simulink model "QC_model"  (R2020a)
settings: Solver=ode5  StartTime=0.0  StopTime=10  FixedStep=basic_time_step  RelTol=1e-3  EnableMultiTasking=on
values from neighbouring files (symbols this model uses):
  b_hat_0 = [0;0;0]    [init.m]
  basic_time_step = 0.001    [init.m]
  e_g = [0;0;1]    [init.m]
  e_m = [1;0;0]    [init.m]
  Eul_hat_0 = [0;0;0]    [init.m]
  g = 9.81    [init.m]
  I = 0.025*eye(3)    [init.m]
  I_inv = inv(I)    [init.m]
  IMU_time_step = 0.002    [init.m]
  k1 = 1    [init.m]
  k2 = 1    [init.m]
  k_I = 10    [init.m]
  k_m = 200    [init.m]
  k_P = 5    [init.m]
  kd = [0.8 0 0 ... (first row only)    [init.m]
  KDP = 2    [init.m]
  KDR = 5    [init.m]
  KDY = 5    [init.m]
  ki = 0*[1.45 0 0 ... (first row only)    [init.m]
  kp = [0.7 0 0 ... (first row only)    [init.m]
  KPP = 35    [init.m]
  KPR = 35    [init.m]
  KPY = 35    [init.m]
  m = 1.5    [init.m]
  m0 = m*1    (= 1.5)    [init.m]
  max_pitch = sin(15*pi/180)    [init.m]
  max_roll = sin(15*pi/180)    [init.m]
  omega_0 = [0 0 0]    [init.m]
  omega_bias = 0*[0.01;-0.005;0.005]    [init.m]
  p_0 = [0 0 0]    [init.m]
  R_0 = eye(3)    [init.m]
  T_act_inv = inv(T_act)    [init.m]
  V_0 = [0 0 0]    [init.m]
  VICON_time_step = 0.016    [init.m]
  w_0 = 0*[1 1 1 1]    [init.m]
  w_max = [inf inf inf inf].^2    [init.m]
  w_min = [0 0 0 0]    [init.m]
undefined symbols (not defined in the file or in its folder): DiscIntNeverNeededParam, q_0
libraries: cstblocks x3, vrlib x2, simulink x1
settings Model: Creator=robu_pa  LastModifiedBy=RyllM
settings DataIOCC: LimitDataPoints=on  SaveFormat=Array  SignalLoggingSaveFormat=ModelDataLogs  ReturnWorkspaceOutputs=off
settings OptimizationCC: ExpressionDepthLimit=2147483647  LifeSpan=inf
settings DebuggingCC: UnderspecifiedInitializationDetection=Classic  MergeDetectMultiDrivingBlocksExec=none  SolverPrmCheckMsg=warning  FcnCallInpInsideContextMsg=warning  StateNameClashWarn=warning  SFUnexpectedBacktrackingDiag=warning  SFNoUnconditionalDefaultTransitionDiag=warning  SFExecutionAtInitializationDiag=none  ArithmeticOperatorsInVariantConditions=warning
settings HardwareCC: ProdBitPerPointer=32  ProdBitPerSizeT=32  ProdBitPerPtrDiffT=32  ProdLargestAtomicFloat=None  ProdIntDivRoundTo=Undefined  ProdEndianess=Unspecified  ProdWordSize=32  ProdHWDeviceType=32-bit Generic
settings ModelReferenceCC: PropagateSignalLabelsOutOfModel=off
settings SFSimCC: SimUseLocalCustomCode=off  CustomCodeUndefinedFunction=UseInterfaceOnly
settings RTWCC: Description=Linux Soft Real-Time Target  SystemTargetFile=lnx.tlc  MakeCommand=make_lnx  TemplateMakefile=lnx_unix.tmf  RTWUseLocalCustomCode=off
settings CodeAppCC: StateflowObjectComments=on
settings STFCustomTargetCC: ModelReferenceCompliant=off  MatFileLogging=on  CPPClassGenCompliant=on  GRTInterface=on  SystemTargetFile=lnx.tlc
settings GRTTargetCC: TargetLangStandard=C89/C90 (ANSI)  ModelReferenceCompliant=off  ParMdlRefBuildCompliant=off  CompOptLevelCompliant=off  ConcurrentExecutionCompliant=off  CombineOutputUpdateFcns=off  GRTInterface=on  UseToolchainInfoCompliant=off  ExtModeMexFile=noextcomm
settings ConfigComp: CovMetricSettings=dw  CovHtmlReporting=on  CovSaveCumulativeToWorkspaceVar=on  CovSaveSingleToWorkspaceVar=on  CovExternalEMLEnable=off

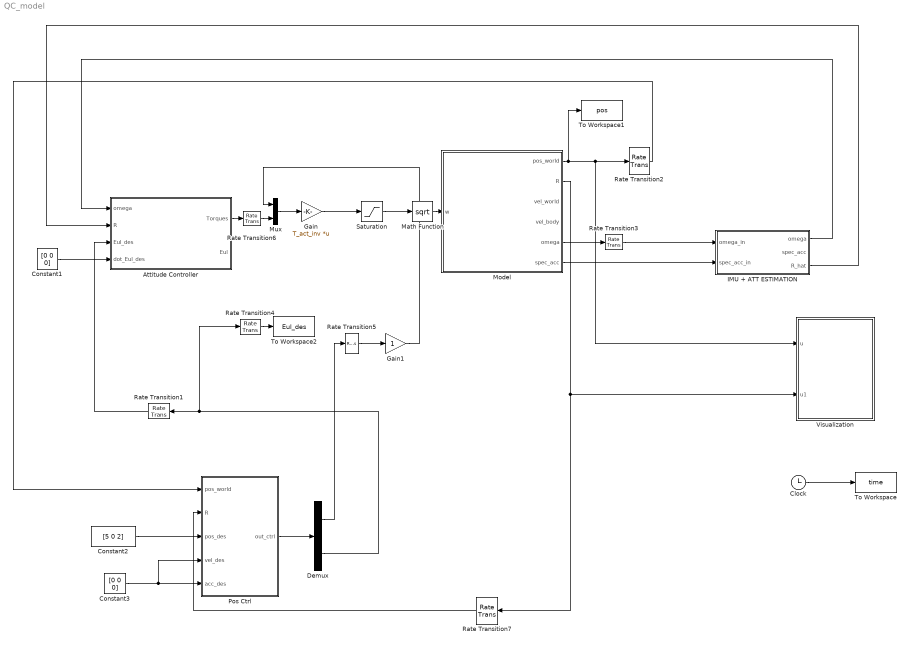
== system QC_model ==
  Attitude Controller : Subsystem  TreatAsAtomicUnit=on  SystemSampleTime=IMU_time_step
  Clock : Clock
  Constant1 : Constant  Value=[0 0 0]
  Constant2 : Constant  Value=[5 0 2]
  Constant3 : Constant  Value=[0 0 0]
  Demux : Demux  Outputs=[1 3]
  Gain : Gain  Gain=T_act_inv  Multiplication=Matrix(K*u)
  Gain1 : Gain
  IMU + ATT ESTIMATION : Subsystem  TreatAsAtomicUnit=on  SystemSampleTime=IMU_time_step
  Math Function : Math  Operator=sqrt  SignedPower=on  SaturateOnIntegerOverflow=on
  Model : Subsystem
  Mux : Mux  Inputs=2
  Pos Ctrl : Subsystem  TreatAsAtomicUnit=on  SystemSampleTime=VICON_time_step
  Rate Transition{1..7} (7 alike) : RateTransition
  Saturation : Saturate  UpperLimit=w_max  LowerLimit=w_min
  To Workspace : ToWorkspace  VariableName=time  SampleTime=-1
  To Workspace1 : ToWorkspace  VariableName=pos  SampleTime=-1
  To Workspace2 : ToWorkspace  VariableName=Eul_des  SampleTime=basic_time_step
  Visualization : Subsystem
  wires:
  Gain/1 -> Saturation/1
  Model/1(pos_world) -> To Workspace1/1, Visualization/1(u), Rate Transition2/1
  Model/6(spec_acc) -> IMU + ATT ESTIMATION/2(spec_acc_in)
  Model/5(omega) -> Rate Transition3/1
  Mux/1 -> Gain/1
  Attitude Controller/1(Torques) -> Rate Transition6/1
  Constant1/1 -> Attitude Controller/4(dot_Eul_des)
  Math Function/1 -> Model/1(w)
  Saturation/1 -> Math Function/1
  Rate Transition2/1 -> Pos Ctrl/1(pos_world)
  Demux/2 -> Rate Transition1/1, Rate Transition4/1
  Constant3/1 -> Pos Ctrl/5(acc_des), Pos Ctrl/4(vel_des)
  Pos Ctrl/1(out_ctrl) -> Demux/1
  Demux/1 -> Rate Transition5/1
  Rate Transition5/1 -> Gain1/1
  Gain1/1 -> Mux/1
  Rate Transition1/1 -> Attitude Controller/3(Eul_des)
  Model/2(R) -> Rate Transition7/1, Visualization/2(u1)
  Rate Transition6/1 -> Mux/2
  Rate Transition3/1 -> IMU + ATT ESTIMATION/1(omega_in)
  Rate Transition4/1 -> To Workspace2/1
  IMU + ATT ESTIMATION/1(omega) -> Attitude Controller/1(omega)
  IMU + ATT ESTIMATION/3(R_hat) -> Attitude Controller/2(R)
  Constant2/1 -> Pos Ctrl/3(pos_des)
  Rate Transition7/1 -> Pos Ctrl/2(R)
  Clock/1 -> To Workspace/1

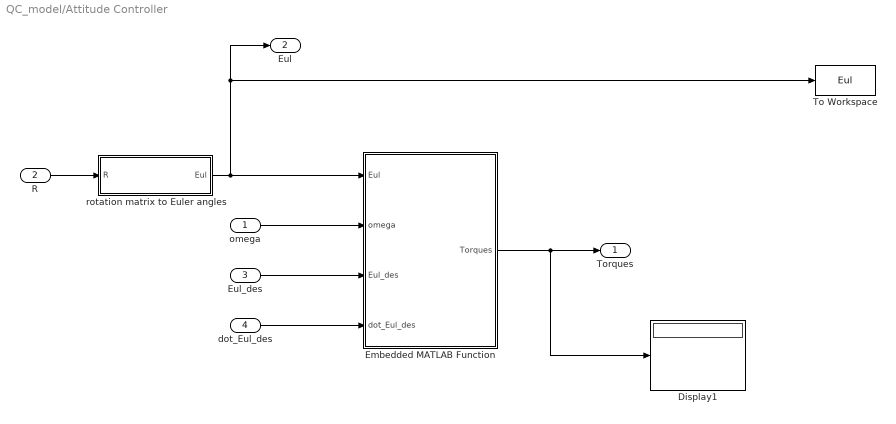
== system QC_model/Attitude Controller ==
  omega : Inport
  R : Inport  Port=2
  Eul_des : Inport  Port=3
  dot_Eul_des : Inport  Port=4
  Display1 : Display
  Embedded MATLAB Function : MATLAB Function  TreatAsAtomicUnit=on
  To Workspace : ToWorkspace  VariableName=Eul  SampleTime=-1
  rotation matrix to Euler angles : MATLAB Function  TreatAsAtomicUnit=on
  Torques : Outport  VectorParamsAs1DForOutWhenUnconnected=off
  Eul : Outport  Port=2  VectorParamsAs1DForOutWhenUnconnected=off
  wires:
  R/1 -> rotation matrix to Euler angles/1(R)
  rotation matrix to Euler angles/1(Eul) -> Embedded MATLAB Function/1(Eul), Eul/1, To Workspace/1
  omega/1 -> Embedded MATLAB Function/2(omega)
  Eul_des/1 -> Embedded MATLAB Function/3(Eul_des)
  dot_Eul_des/1 -> Embedded MATLAB Function/4(dot_Eul_des)
  Embedded MATLAB Function/1(Torques) -> Torques/1, Display1/1

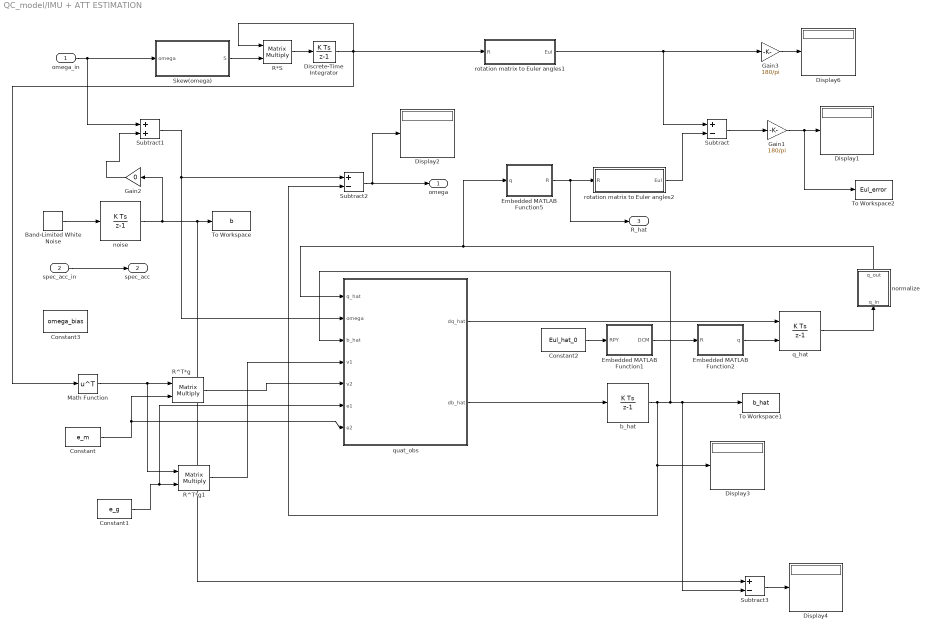
== system QC_model/IMU + ATT ESTIMATION ==
  omega_in : Inport
  spec_acc_in : Inport  Port=2
  Band-Limited White Noise : simulink/Sources/Band-Limited White Noise  Cov=[.0001 .0001 .0001]  Ts=IMU_time_step  seed=[23341 453 123]
  Constant : Constant  Value=e_m
  Constant1 : Constant  Value=e_g
  Constant2 : Constant  Value=Eul_hat_0
  Constant3 : Constant  Value=omega_bias
  Discrete-Time Integrator : DiscreteIntegrator  InitialCondition=R_0  SampleTime=-1  ICPrevOutput=DiscIntNeverNeededParam  ICPrevScaledInput=DiscIntNeverNeededParam
  Display{1..4,6} (5 alike) : Display
  Embedded MATLAB Function1 : MATLAB Function  TreatAsAtomicUnit=on
  Embedded MATLAB Function2 : MATLAB Function  TreatAsAtomicUnit=on
  Embedded MATLAB Function5 : MATLAB Function  TreatAsAtomicUnit=on
  Gain1 : Gain  Gain=180/pi
  Gain2 : Gain  Gain=0
  Gain3 : Gain  Gain=180/pi
  Math Function : Math  Operator=transpose  SignedPower=on  SaturateOnIntegerOverflow=on
  R*S : Product  Multiplication=Matrix(*)  RndMeth=Zero
  R^T*g : Product  Multiplication=Matrix(*)  RndMeth=Zero
  R^T*g1 : Product  Multiplication=Matrix(*)  RndMeth=Zero
  Skew(omega) : MATLAB Function  TreatAsAtomicUnit=on
  Subtract : Sum  Inputs=+-
  Subtract1 : Sum
  Subtract2 : Sum  Inputs=+-
  Subtract3 : Sum  Inputs=+-
  To Workspace : ToWorkspace  VariableName=b  SampleTime=-1
  To Workspace1 : ToWorkspace  VariableName=b_hat  SampleTime=-1
  To Workspace2 : ToWorkspace  VariableName=Eul_error  SampleTime=-1
  b_hat : DiscreteIntegrator  InitialCondition=b_hat_0  SampleTime=-1  ICPrevOutput=DiscIntNeverNeededParam  ICPrevScaledInput=DiscIntNeverNeededParam
  noise : DiscreteIntegrator  InitialCondition=b_hat_0  SampleTime=-1  ICPrevOutput=DiscIntNeverNeededParam  ICPrevScaledInput=DiscIntNeverNeededParam
  normalize : MATLAB Function  TreatAsAtomicUnit=on
  q_hat : DiscreteIntegrator  InitialConditionSource=external  InitialCondition=q_0  SampleTime=-1  ICPrevOutput=DiscIntNeverNeededParam  ICPrevScaledInput=DiscIntNeverNeededParam
  quat_obs : MATLAB Function  TreatAsAtomicUnit=on
  rotation matrix to Euler angles1 : MATLAB Function  TreatAsAtomicUnit=on
  rotation matrix to Euler angles2 : MATLAB Function  TreatAsAtomicUnit=on
  omega : Outport  VectorParamsAs1DForOutWhenUnconnected=off
  spec_acc : Outport  Port=2  VectorParamsAs1DForOutWhenUnconnected=off
  R_hat : Outport  Port=3  VectorParamsAs1DForOutWhenUnconnected=off
  wires:
  spec_acc_in/1 -> spec_acc/1
  omega_in/1 -> Skew(omega)/1(omega), Subtract1/1
  R*S/1 -> Discrete-Time Integrator/1
  Discrete-Time Integrator/1 -> Math Function/1, R*S/1, rotation matrix to Euler angles1/1(R)
  Skew(omega)/1(S) -> R*S/2
  rotation matrix to Euler angles1/1(Eul) -> Gain3/1, Subtract/1
  Gain3/1 -> Display6/1
  Math Function/1 -> R^T*g/1, R^T*g1/1
  Constant/1 -> R^T*g/2, quat_obs/7(e2)
  Constant2/1 -> Embedded MATLAB Function1/1(RPY)
  Embedded MATLAB Function1/1(DCM) -> Embedded MATLAB Function2/1(R)
  Embedded MATLAB Function2/1(q) -> q_hat/2
  quat_obs/1(dq_hat) -> q_hat/1
  quat_obs/2(db_hat) -> b_hat/1
  q_hat/1 -> normalize/1(q_in)
  b_hat/1 -> Display3/1, Subtract2/2, quat_obs/3(b_hat), To Workspace1/1, Subtract3/2
  Constant1/1 -> R^T*g1/2, quat_obs/6(e1)
  R^T*g/1 -> quat_obs/5(v2)
  R^T*g1/1 -> quat_obs/4(v1)
  Embedded MATLAB Function5/1(R) -> rotation matrix to Euler angles2/1(R), R_hat/1
  rotation matrix to Euler angles2/1(Eul) -> Subtract/2
  Subtract/1 -> Gain1/1
  Gain1/1 -> Display1/1, To Workspace2/1
  Subtract1/1 -> Subtract2/1, quat_obs/2(omega)
  Gain2/1 -> Subtract1/2
  Subtract2/1 -> Display2/1, omega/1
  normalize/1(q_out) -> Embedded MATLAB Function5/1(q), quat_obs/1(q_hat)
  Band-Limited White Noise/1 -> noise/1
  noise/1 -> Gain2/1, To Workspace/1, Subtract3/1
  Subtract3/1 -> Display4/1

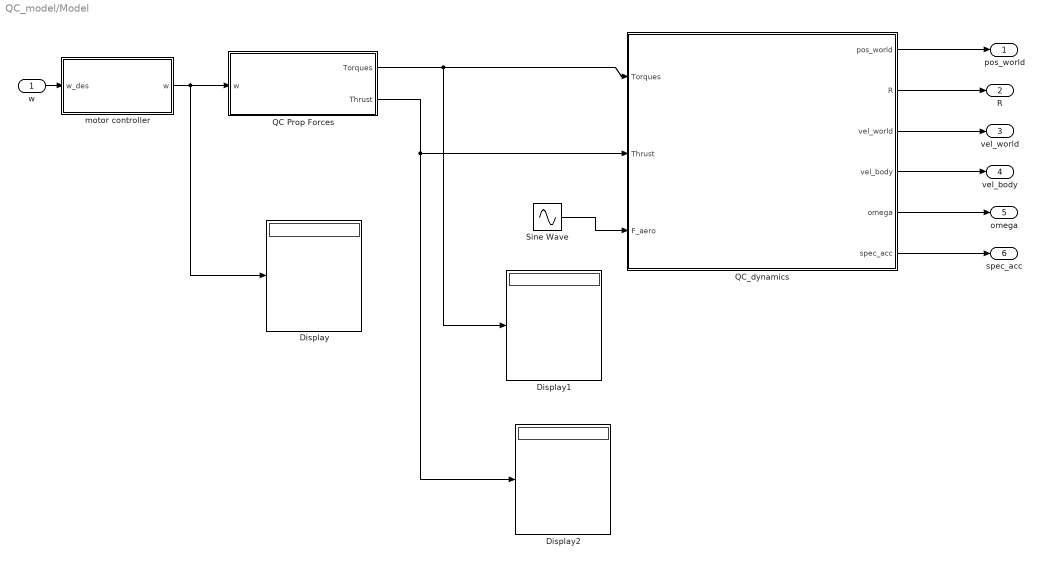
== system QC_model/Model ==
  w : Inport
  Display : Display
  Display1 : Display
  Display2 : Display
  QC Prop Forces : MATLAB Function  TreatAsAtomicUnit=on
  QC_dynamics : Subsystem
  Sine Wave : Sin  Amplitude=[0; 0; 0]  SampleTime=0
  motor controller : Subsystem
  pos_world : Outport  VectorParamsAs1DForOutWhenUnconnected=off
  R : Outport  Port=2  VectorParamsAs1DForOutWhenUnconnected=off
  vel_world : Outport  Port=3  VectorParamsAs1DForOutWhenUnconnected=off
  vel_body : Outport  Port=4  VectorParamsAs1DForOutWhenUnconnected=off
  omega : Outport  Port=5  VectorParamsAs1DForOutWhenUnconnected=off
  spec_acc : Outport  Port=6  VectorParamsAs1DForOutWhenUnconnected=off
  wires:
  QC Prop Forces/1(Torques) -> QC_dynamics/1(Torques), Display1/1
  QC Prop Forces/2(Thrust) -> QC_dynamics/2(Thrust), Display2/1
  w/1 -> motor controller/1(w_des)
  QC_dynamics/1(pos_world) -> pos_world/1
  QC_dynamics/2(R) -> R/1
  QC_dynamics/3(vel_world) -> vel_world/1
  QC_dynamics/4(vel_body) -> vel_body/1
  QC_dynamics/5(omega) -> omega/1
  QC_dynamics/6(spec_acc) -> spec_acc/1
  motor controller/1(w) -> QC Prop Forces/1(w), Display/1
  Sine Wave/1 -> QC_dynamics/3(F_aero)

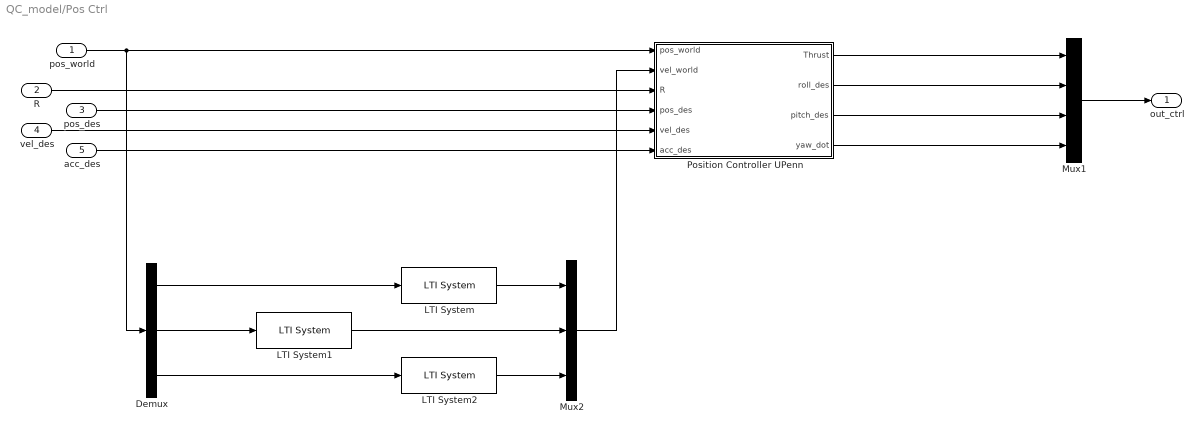
== system QC_model/Pos Ctrl ==
  pos_world : Inport
  R : Inport  Port=2
  pos_des : Inport  Port=3
  vel_des : Inport  Port=4
  acc_des : Inport  Port=5
  Demux : Demux  Outputs=3
  LTI System : cstblocks/LTI System  sys=fil_vel  IC=[]
  LTI System1 : cstblocks/LTI System  sys=fil_vel  IC=[]
  LTI System2 : cstblocks/LTI System  sys=fil_vel  IC=[]
  Mux1 : Mux
  Mux2 : Mux  Inputs=3
  Position Controller UPenn : Subsystem  SystemSampleTime=VICON_time_step
  out_ctrl : Outport  VectorParamsAs1DForOutWhenUnconnected=off
  wires:
  pos_world/1 -> Position Controller UPenn/1(pos_world), Demux/1
  R/1 -> Position Controller UPenn/3(R)
  pos_des/1 -> Position Controller UPenn/4(pos_des)
  vel_des/1 -> Position Controller UPenn/5(vel_des)
  acc_des/1 -> Position Controller UPenn/6(acc_des)
  Position Controller UPenn/1(Thrust) -> Mux1/1
  Position Controller UPenn/2(roll_des) -> Mux1/2
  Position Controller UPenn/3(pitch_des) -> Mux1/3
  Position Controller UPenn/4(yaw_dot) -> Mux1/4
  Demux/1 -> LTI System/1
  LTI System/1 -> Mux2/1
  Demux/2 -> LTI System1/1
  LTI System1/1 -> Mux2/2
  Demux/3 -> LTI System2/1
  LTI System2/1 -> Mux2/3
  Mux2/1 -> Position Controller UPenn/2(vel_world)
  Mux1/1 -> out_ctrl/1

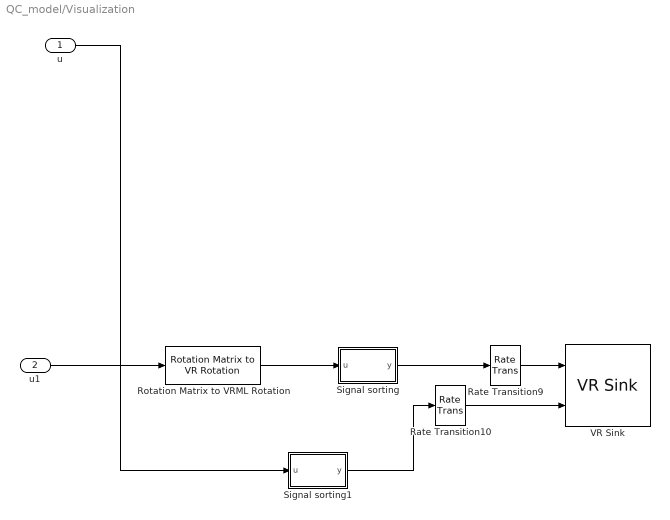
== system QC_model/Visualization ==
  u : Inport
  u1 : Inport  Port=2
  Rate Transition10 : RateTransition
  Rate Transition9 : RateTransition
  Rotation Matrix to VRML Rotation : vrlib/Utilities/Rotation Matrix to VR Rotation  maxzero=1e-12
      settings: SourceProductBaseCode=SL
  Signal sorting : MATLAB Function  TreatAsAtomicUnit=on
  Signal sorting1 : MATLAB Function  TreatAsAtomicUnit=on
  VR Sink : vrlib/VR Sink  InstantiateOnLoad=on  SampleTime=0.03  ViewEnable=on  RemoteChange=off  RemoteView=off  FieldsWritten=Quad.rotation.4.1.1.double#Quad.translation.3.1.1.double  WorldFileName=Quad.wrl  AutoView=off  VideoDimensions=[]  AllowVariableSize=off
  wires:
  Rate Transition10/1 -> VR Sink/2
  Rotation Matrix to VRML Rotation/1 -> Signal sorting/1(u)
  Rate Transition9/1 -> VR Sink/1
  Signal sorting/1(y) -> Rate Transition9/1
  Signal sorting1/1(y) -> Rate Transition10/1
  u1/1 -> Rotation Matrix to VRML Rotation/1
  u/1 -> Signal sorting1/1(u)

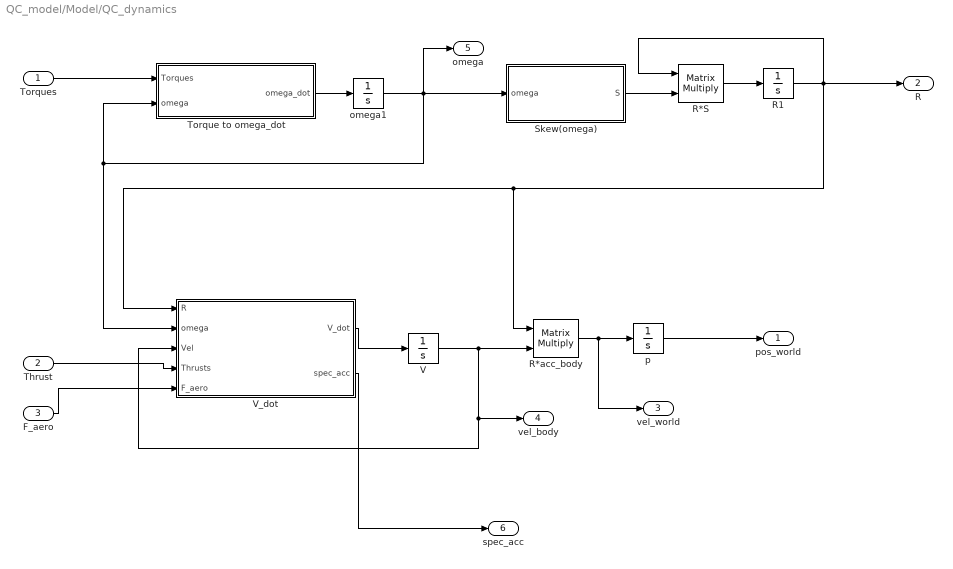
== system QC_model/Model/QC_dynamics ==
  Torques : Inport
  Thrust : Inport  Port=2
  F_aero : Inport  Port=3
  R*S : Product  Multiplication=Matrix(*)  RndMeth=Zero
  R*acc_body : Product  Multiplication=Matrix(*)  RndMeth=Zero
  R1 : Integrator  InitialCondition=R_0
  Skew(omega) : MATLAB Function  TreatAsAtomicUnit=on
  Torque to omega_dot : Subsystem
  V : Integrator  InitialCondition=V_0
  V_dot : Subsystem
  omega1 : Integrator  InitialCondition=omega_0
  p : Integrator  InitialCondition=p_0
  pos_world : Outport  VectorParamsAs1DForOutWhenUnconnected=off
  R : Outport  Port=2  VectorParamsAs1DForOutWhenUnconnected=off
  vel_world : Outport  Port=3  VectorParamsAs1DForOutWhenUnconnected=off
  vel_body : Outport  Port=4  VectorParamsAs1DForOutWhenUnconnected=off
  omega : Outport  Port=5  VectorParamsAs1DForOutWhenUnconnected=off
  spec_acc : Outport  Port=6  VectorParamsAs1DForOutWhenUnconnected=off
  wires:
  V_dot/1(V_dot) -> V/1
  V/1 -> R*acc_body/2, V_dot/3(Vel), vel_body/1
  R*acc_body/1 -> p/1, vel_world/1
  Torque to omega_dot/1(omega_dot) -> omega1/1
  omega1/1 -> V_dot/2(omega), Torque to omega_dot/2(omega), Skew(omega)/1(omega), omega/1
  R*S/1 -> R1/1
  R1/1 -> R*acc_body/1, V_dot/1(R), R/1, R*S/1
  Skew(omega)/1(S) -> R*S/2
  Thrust/1 -> V_dot/4(Thrusts)
  Torques/1 -> Torque to omega_dot/1(Torques)
  p/1 -> pos_world/1
  F_aero/1 -> V_dot/5(F_aero)
  V_dot/2(spec_acc) -> spec_acc/1

== system QC_model/Model/motor controller ==
  w_des : Inport
  Gain : Gain  Gain=k_m
  Integrator : Integrator  InitialCondition=w_0
  Subtract : Sum  Inputs=+-
  w : Outport  VectorParamsAs1DForOutWhenUnconnected=off
  wires:
  Integrator/1 -> w/1, Subtract/2
  Gain/1 -> Integrator/1
  Subtract/1 -> Gain/1
  w_des/1 -> Subtract/1

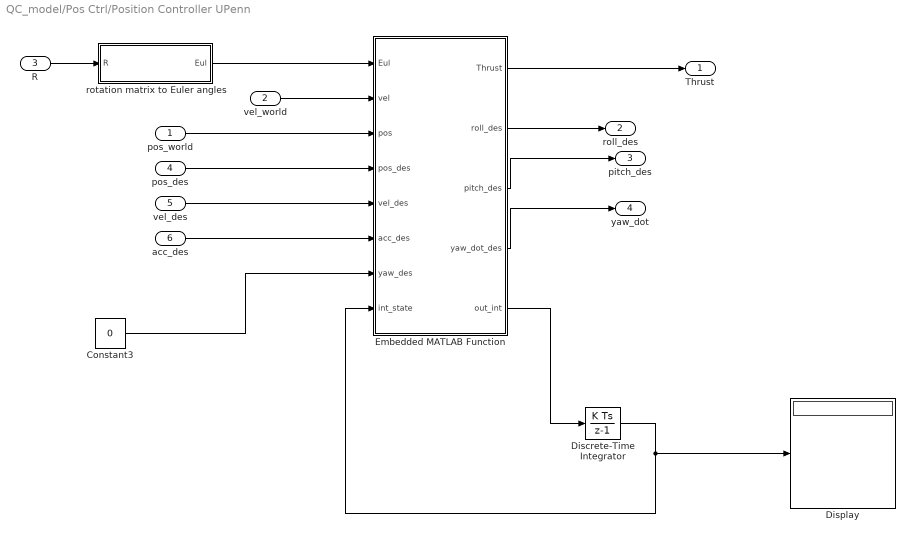
== system QC_model/Pos Ctrl/Position Controller UPenn ==
  pos_world : Inport
  vel_world : Inport  Port=2
  R : Inport  Port=3
  pos_des : Inport  Port=4
  vel_des : Inport  Port=5
  acc_des : Inport  Port=6
  Constant3 : Constant  Value=0
  Discrete-Time Integrator : DiscreteIntegrator  InitialCondition=[0 0 0]  SampleTime=-1  ICPrevOutput=DiscIntNeverNeededParam  ICPrevScaledInput=DiscIntNeverNeededParam
  Display : Display
  Embedded MATLAB Function : MATLAB Function  TreatAsAtomicUnit=on
  rotation matrix to Euler angles : MATLAB Function  TreatAsAtomicUnit=on
  Thrust : Outport  VectorParamsAs1DForOutWhenUnconnected=off
  roll_des : Outport  Port=2  VectorParamsAs1DForOutWhenUnconnected=off
  pitch_des : Outport  Port=3  VectorParamsAs1DForOutWhenUnconnected=off
  yaw_dot : Outport  Port=4  VectorParamsAs1DForOutWhenUnconnected=off
  wires:
  R/1 -> rotation matrix to Euler angles/1(R)
  rotation matrix to Euler angles/1(Eul) -> Embedded MATLAB Function/1(Eul)
  vel_world/1 -> Embedded MATLAB Function/2(vel)
  pos_world/1 -> Embedded MATLAB Function/3(pos)
  Embedded MATLAB Function/1(Thrust) -> Thrust/1
  pos_des/1 -> Embedded MATLAB Function/4(pos_des)
  vel_des/1 -> Embedded MATLAB Function/5(vel_des)
  acc_des/1 -> Embedded MATLAB Function/6(acc_des)
  Constant3/1 -> Embedded MATLAB Function/7(yaw_des)
  Embedded MATLAB Function/2(roll_des) -> roll_des/1
  Embedded MATLAB Function/3(pitch_des) -> pitch_des/1
  Embedded MATLAB Function/4(yaw_dot_des) -> yaw_dot/1
  Embedded MATLAB Function/5(out_int) -> Discrete-Time Integrator/1
  Discrete-Time Integrator/1 -> Embedded MATLAB Function/8(int_state), Display/1

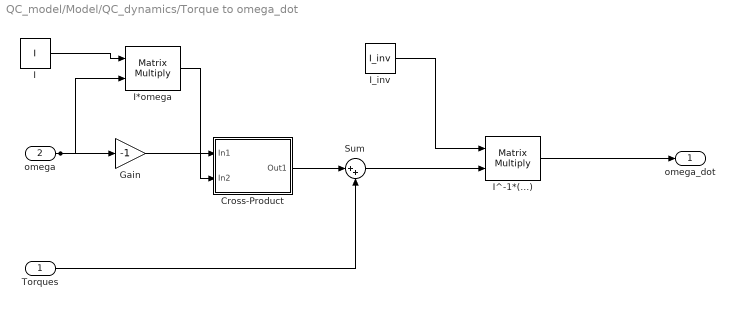
== system QC_model/Model/QC_dynamics/Torque to omega_dot ==
  Torques : Inport
  omega : Inport  Port=2
  Cross-Product : Subsystem
  Gain : Gain  Gain=-1
  I : Constant  Value=I
  I*omega : Product  Multiplication=Matrix(*)  RndMeth=Zero
  I^-1*(...) : Product  Multiplication=Matrix(*)  RndMeth=Zero
  I_inv : Constant  Value=I_inv
  Sum : Sum  Inputs=|++
  omega_dot : Outport  VectorParamsAs1DForOutWhenUnconnected=off
  wires:
  omega/1 -> I*omega/2, Gain/1
  I/1 -> I*omega/1
  I*omega/1 -> Cross-Product/2(In2)
  I^-1*(...)/1 -> omega_dot/1
  Torques/1 -> Sum/2
  Sum/1 -> I^-1*(...)/2
  Gain/1 -> Cross-Product/1(In1)
  Cross-Product/1(Out1) -> Sum/1
  I_inv/1 -> I^-1*(...)/1

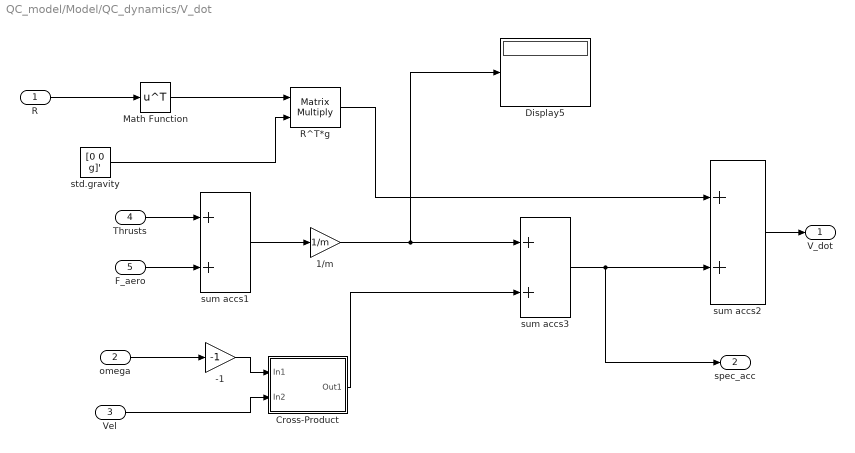
== system QC_model/Model/QC_dynamics/V_dot ==
  R : Inport
  omega : Inport  Port=2
  Vel : Inport  Port=3
  Thrusts : Inport  Port=4
  F_aero : Inport  Port=5
  -1 : Gain  Gain=-1
  1/m : Gain  Gain=1/m
  Cross-Product : Subsystem
  Display5 : Display
  Math Function : Math  Operator=transpose  SignedPower=on  SaturateOnIntegerOverflow=on
  R^T*g : Product  Multiplication=Matrix(*)  RndMeth=Zero
  std.gravity : Constant  Value=[0 0 g]'
  sum accs1 : Sum
  sum accs2 : Sum
  sum accs3 : Sum
  V_dot : Outport  VectorParamsAs1DForOutWhenUnconnected=off
  spec_acc : Outport  Port=2  VectorParamsAs1DForOutWhenUnconnected=off
  wires:
  omega/1 -> -1/1
  Vel/1 -> Cross-Product/2(In2)
  R/1 -> Math Function/1
  Math Function/1 -> R^T*g/1
  std.gravity/1 -> R^T*g/2
  R^T*g/1 -> sum accs2/1
  sum accs2/1 -> V_dot/1
  1/m/1 -> sum accs3/1, Display5/1
  -1/1 -> Cross-Product/1(In1)
  Cross-Product/1(Out1) -> sum accs3/2
  Thrusts/1 -> sum accs1/1
  sum accs1/1 -> 1/m/1
  F_aero/1 -> sum accs1/2
  sum accs3/1 -> sum accs2/2, spec_acc/1

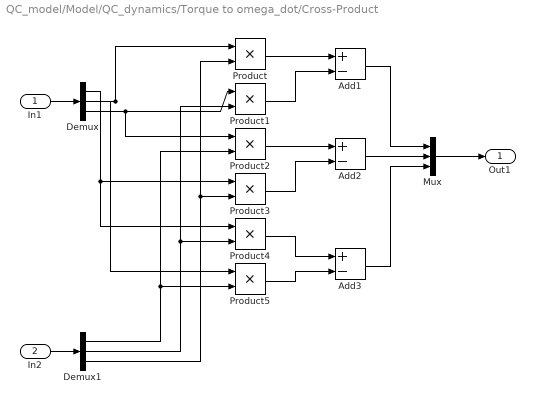
== system QC_model/Model/QC_dynamics/Torque to omega_dot/Cross-Product ==
  In1 : Inport
  In2 : Inport  Port=2
  Add1 : Sum  Inputs=+-
  Add2 : Sum  Inputs=+-
  Add3 : Sum  Inputs=+-
  Demux : Demux  Outputs=3
  Demux1 : Demux  Outputs=3
  Mux : Mux  Inputs=3
  Product{,1..5} (6 alike) : Product  RndMeth=Zero
  Out1 : Outport  VectorParamsAs1DForOutWhenUnconnected=off
  wires:
  In1/1 -> Demux/1
  In2/1 -> Demux1/1
  Mux/1 -> Out1/1
  Add1/1 -> Mux/1
  Add2/1 -> Mux/2
  Add3/1 -> Mux/3
  Demux/2 -> Product/1, Product5/1
  Demux1/3 -> Product/2, Product3/2
  Demux/3 -> Product1/1, Product2/1
  Demux1/2 -> Product1/2, Product4/2
  Demux/1 -> Product3/1, Product4/1
  Demux1/1 -> Product2/2, Product5/2
  Product/1 -> Add1/1
  Product1/1 -> Add1/2
  Product2/1 -> Add2/1
  Product3/1 -> Add2/2
  Product4/1 -> Add3/1
  Product5/1 -> Add3/2

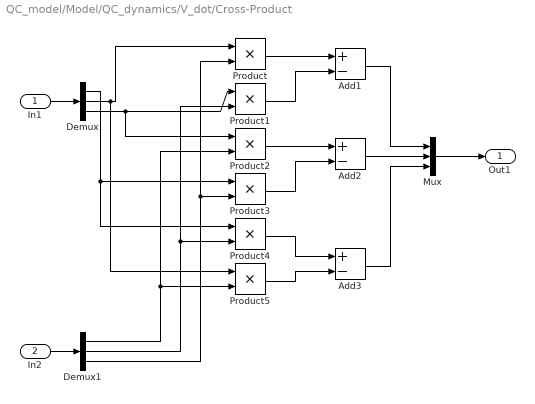
== system QC_model/Model/QC_dynamics/V_dot/Cross-Product ==
  In1 : Inport
  In2 : Inport  Port=2
  Add1 : Sum  Inputs=+-
  Add2 : Sum  Inputs=+-
  Add3 : Sum  Inputs=+-
  Demux : Demux  Outputs=3
  Demux1 : Demux  Outputs=3
  Mux : Mux  Inputs=3
  Product{,1..5} (6 alike) : Product  RndMeth=Zero
  Out1 : Outport  VectorParamsAs1DForOutWhenUnconnected=off
  wires:
  In1/1 -> Demux/1
  In2/1 -> Demux1/1
  Mux/1 -> Out1/1
  Add1/1 -> Mux/1
  Add2/1 -> Mux/2
  Add3/1 -> Mux/3
  Demux/2 -> Product/1, Product5/1
  Demux1/3 -> Product/2, Product3/2
  Demux/3 -> Product1/1, Product2/1
  Demux1/2 -> Product1/2, Product4/2
  Demux/1 -> Product3/1, Product4/1
  Demux1/1 -> Product2/2, Product5/2
  Product/1 -> Add1/1
  Product1/1 -> Add1/2
  Product2/1 -> Add2/1
  Product3/1 -> Add2/2
  Product4/1 -> Add3/1
  Product5/1 -> Add3/2

== matlab function QC_model/Visualization/Signal sorting ==
  data: u input; y output
function y = fcn(u)

y = [u(2) u(2) u(2) u(4)];

== matlab function QC_model/IMU + ATT ESTIMATION/Embedded MATLAB Function1 ==
  data: RPY input; DCM output
function DCM = BF2IF(RPY)
% This block supports the Embedded MATLAB subset.
% See the help menu for details. 

r = RPY(1);
p = RPY(2);
y = RPY(3);
RPYrot = [ cos(y)*cos(p)  cos(y)*sin(p)*sin(r)-sin(y)*cos(r)  cos(y)*sin(p)*cos(r)+sin(y)*sin(r);
          sin(y)*cos(p)  sin(y)*sin(p)*sin(r)+cos(y)*cos(r)  sin(y)*sin(p)*cos(r)-cos(y)*sin(r);
             -sin(p)                  cos(p)*sin(r)                      cos(p)*cos(r)];

DCM = RPYrot;

== matlab function QC_model/IMU + ATT ESTIMATION/Embedded MATLAB Function2 ==
  data: R input; q output
function q = R2q(R)
% This block supports the Embedded MATLAB subset.
% See the help menu for details. 


theta=acos( (trace(R)-1)/2 );

if (abs(theta)>.1*pi/180)
    
    a=1/(2*sin(theta))*[R(3,2)-R(2,3);
        R(1,3)-R(3,1);
        R(2,1)-R(1,2)];
    
else
        
    a=[0;0;0];
    
end


q=[cos(theta/2);sin(theta/2)*a];

q=q/norm(q);

== matlab function QC_model/IMU + ATT ESTIMATION/Embedded MATLAB Function5 ==
  data: R output; q input
function R = q2R(q)
% This block supports the Embedded MATLAB subset.
% See the help menu for details. 


s=q(1);
v=q(2:4);

R=eye(3)+2*s*skew(v)+2*skew(v)*skew(v);






function S = skew(omega)
% This block supports the Embedded MATLAB subset.
% See the help menu for details. 
S = [0 -omega(3) omega(2);
 omega(3) 0 -omega(1);
 -omega(2) omega(1) 0];

== matlab function QC_model/IMU + ATT ESTIMATION/rotation matrix to Euler angles2 ==
  data: R input; Eul output
function Eul = eulerangles(R)
% This block supports an embeddable subset of the MATLAB language.
% See the help menu for details. 

Roll = atan2(R(3,2),R(3,3));
Pitch = atan2(-R(3,1),sqrt(R(3,2)^2+R(3,3)^2));
Yaw = atan2(R(2,1),R(1,1));


Eul = [Roll; Pitch; Yaw];

== matlab function QC_model/IMU + ATT ESTIMATION/normalize ==
  data: q_in input; q_out output
function q_out = skew(q_in)
% This block supports the Embedded MATLAB subset.
% See the help menu for details. 

q_out=q_in/norm(q_in);

== matlab function QC_model/IMU + ATT ESTIMATION/quat_obs ==
  data: q_hat input; omega input; dq_hat output; b_hat input; v1 input; v2 input; db_hat output; e1 input; e2 input; k1 parameter; k2 parameter; k_P parameter; k_I parameter
function [dq_hat, db_hat] = quat_obs(q_hat, omega, b_hat, v1, v2, e1, e2, k1, k2, k_P, k_I)
% This block supports the Embedded MATLAB subset.
% See the help menu for details. 

R_hat=q2R(q_hat);

v1_hat=R_hat'*e1;
v2_hat=R_hat'*e2;

v1=v1/norm(v1);
v2=v2/norm(v2);


wmes=vex(-(k1/2*(v1*v1_hat' - v1_hat*v1') + k2/2*(v2*v2_hat' - v2_hat*v2')));

dq_hat=diff_q(q_hat, omega-b_hat+k_P*wmes);

db_hat=-k_I*wmes;







function dq=diff_q(q, omega)

pomega=[0;omega];


s1=q(1);
s2=pomega(1);

v1=q(2:4);
v2=pomega(2:4);

dq=.5*[s1*s2-v1'*v2;
    s1*v2+s2*v1+cross(v1,v2)];






function R = q2R(q)
% This block supports the Embedded MATLAB subset.
% See the help menu for details. 


s=q(1);
v=q(2:4);

R=eye(3)+2*s*skew(v)+2*skew(v)*skew(v);



function v=vex(tmp)

 v=[tmp(3,2);
    tmp(1,3);
    tmp(2,1)];



function S = skew(omega)
% This block supports the Embedded MATLAB subset.
% See the help menu for details. 
S = [0 -omega(3) omega(2);
 omega(3) 0 -omega(1);
 -omega(2) omega(1) 0];

== matlab function QC_model/Visualization/Signal sorting1 ==
  data: u input; y output
function y = fcn(u)

y = [u(1) u(3) -u(2)];

== matlab function QC_model/Model/QC_dynamics/Skew(omega) ==
  data: omega input; S output
function S = skew(omega)
% This block supports the Embedded MATLAB subset.
% See the help menu for details. 
S = [0 -omega(3) omega(2);
 omega(3) 0 -omega(1);
 -omega(2) omega(1) 0];

== matlab function QC_model/Attitude Controller/rotation matrix to Euler angles ==
  data: R input; Eul output
function Eul = eulerangles(R)
% This block supports an embeddable subset of the MATLAB language.
% See the help menu for details. 

Roll = atan2(R(3,2),R(3,3));
Pitch = atan2(-R(3,1),sqrt(R(3,2)^2+R(3,3)^2));
Yaw = atan2(R(2,1),R(1,1));


Eul = [Roll; Pitch; Yaw];

== matlab function QC_model/Attitude Controller/Embedded MATLAB Function ==
  data: Eul input; Torques output; omega input; Eul_des input; dot_Eul_des input; KDR parameter; KPR parameter; KDP parameter; KPP parameter; KDY parameter; KPY parameter
function Torques  = fcn(Eul, omega, Eul_des, dot_Eul_des, KDR, KPR, KDP, KPP, KDY, KPY)
% This block supports the Embedded MATLAB subset.
% See the help menu for details. 

Torques=[0;0;0];

r = Eul(1);
p = Eul(2);
y = Eul(3);


T = [1      tan(p)*sin(r) tan(p)*cos(r);
    0       cos(r)  -sin(r);
    0       sin(r)/cos(p)   cos(r)/cos(p)];


% T=eye(3);

dot_Eul = T*omega;

dot_r = dot_Eul(1);
dot_p = dot_Eul(2);
dot_y = dot_Eul(3);

% U=I*inv(T)*([ KDR * (0 - dot_r) + KPR * (roll_des - r); KDP * (0 - dot_p) + KPP * (pitch_des - p) ; KPY * (yaw_dot_des - dot_y) ]);


Torques(1) = KDR * (dot_Eul_des(1) - dot_r) + KPR * (Eul_des(1) - r);
Torques(2) = KDP * (dot_Eul_des(2) - dot_p) + KPP * (Eul_des(2) - p);
Torques(3) = KDY * (dot_Eul_des(3) - dot_y) + KPY * (Eul_des(3) - y);

== matlab function QC_model/Model/QC Prop Forces ==
  data: w input; Torques output; Thrust output; T_act parameter
function [Torques, Thrust]= fcn(w, T_act)
% This block supports the Embedded MATLAB subset.
% See the help menu for details. 



res=T_act*(w.^2);

Thrust=[0;0;res(1)];

Torques=res(2:4);

== matlab function QC_model/Pos Ctrl/Position Controller UPenn/Embedded MATLAB Function ==
  data: Eul input; Thrust output; roll_des output; pitch_des output; yaw_dot_des output; vel input; pos input; pos_des input; vel_des input; acc_des input; yaw_des input; int_state input; m0 parameter; g parameter; out_int output; VICON_time_step parameter; kp parameter; kd parameter; ki parameter; max_roll parameter; max_pitch parameter
function [Thrust, roll_des, pitch_des, yaw_dot_des, out_int]  = fcn(Eul, vel, pos, pos_des, vel_des, acc_des, yaw_des, int_state, m0, g, VICON_time_step, kp, kd, ki, max_roll, max_pitch)
% This block supports the Embedded MATLAB subset.
% See the help menu for details. 



r = Eul(1);
p = Eul(2);
y = Eul(3);



acc_des=-kd*vel+kp*(pos_des-pos)+int_state;


out_int=ki*(pos_des-pos);


Thrust=-m0*g+acc_des(3);

roll_des=(-sin(y)*acc_des(1)+cos(y)*acc_des(2))/g;
pitch_des=-(cos(y)*acc_des(1)+sin(y)*acc_des(2))/g;

yaw_dot_des=0;




if abs(roll_des)>asin(max_roll)
    roll_des=sign(roll_des)*asin(max_roll);
end




if abs(pitch_des)>asin(max_pitch)
    pitch_des=sign(pitch_des)*asin(max_pitch);
end




% if (Thrust>-5)
%     Thrust=-5;
% end
% 
% 
% if (Thrust<-2*m0*g+5)
%     Thrust=-2*m0*g+5;
% end

== matlab function QC_model/Pos Ctrl/Position Controller UPenn/rotation matrix to Euler angles ==
  data: R input; Eul output
function Eul = eulerangles(R)
% This block supports an embeddable subset of the MATLAB language.
% See the help menu for details. 

Roll = atan2(R(3,2),R(3,3));
Pitch = atan2(-R(3,1),sqrt(R(3,2)^2+R(3,3)^2));
Yaw = atan2(R(2,1),R(1,1));


Eul = [Roll; Pitch; Yaw];

== matlab function QC_model/IMU + ATT ESTIMATION/Skew(omega) ==
  data: omega input; S output
function S = skew(omega)
% This block supports the Embedded MATLAB subset.
% See the help menu for details. 
S = [0 -omega(3) omega(2);
 omega(3) 0 -omega(1);
 -omega(2) omega(1) 0];

== matlab function QC_model/IMU + ATT ESTIMATION/rotation matrix to Euler angles1 ==
  data: R input; Eul output
function Eul = eulerangles(R)
% This block supports an embeddable subset of the MATLAB language.
% See the help menu for details. 

Roll = atan2(R(3,2),R(3,3));
Pitch = atan2(-R(3,1),sqrt(R(3,2)^2+R(3,3)^2));
Yaw = atan2(R(2,1),R(1,1));


Eul = [Roll; Pitch; Yaw];
